simulink model "A01274570_ACT_MATLAB_ROBOTDK"  (R2022a)
settings: Solver=ode45  StartTime=0.0  StopTime=60  MaxStep=.2  RelTol=1e-3  EnableMultiTasking=on
PreLoadFcn:
  | clear all
settings Model: Creator=Student  LastModifiedBy=osher
settings SolverCC: AlgebraicLoopSolver=TrustRegion
settings DataIOCC: LimitDataPoints=on  SaveFormat=Array  ReturnWorkspaceOutputs=off
settings OptimizationCC: LifeSpan=inf
settings DebuggingCC: UnconnectedInputMsg=warning  UnconnectedOutputMsg=warning  UnconnectedLineMsg=warning  SFUnexpectedBacktrackingDiag=warning  SFNoUnconditionalDefaultTransitionDiag=warning  SFExecutionAtInitializationDiag=none  SFMachineParentedDataDiag=warning  ArithmeticOperatorsInVariantConditions=warning
settings HardwareCC: ProdBitPerPointer=32  ProdBitPerSizeT=32  ProdBitPerPtrDiffT=32  ProdLargestAtomicFloat=None  ProdIntDivRoundTo=Undefined  ProdEndianess=Unspecified  ProdWordSize=32  ProdHWDeviceType=32-bit Generic
settings ModelReferenceCC: PropagateSignalLabelsOutOfModel=off
settings SFSimCC: SimUseLocalCustomCode=off  CustomCodeUndefinedFunction=UseInterfaceOnly
settings RTWCC: RTWUseLocalCustomCode=off
settings CodeAppCC: StateflowObjectComments=on
settings GRTTargetCC: TargetLangStandard=C89/C90 (ANSI)
settings ConfigComp: CovMetricSettings=dw  CovSaveCumulativeToWorkspaceVar=on  CovSaveSingleToWorkspaceVar=on  CovExternalEMLEnable=off

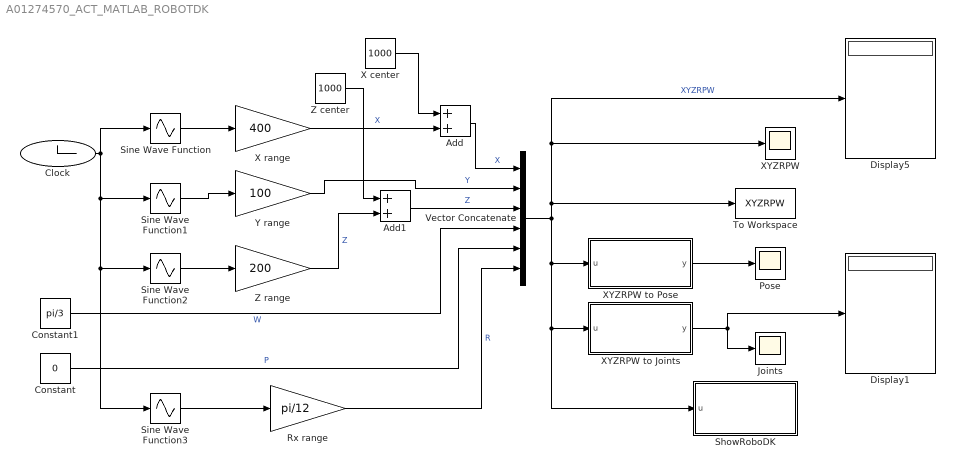
== system A01274570_ACT_MATLAB_ROBOTDK ==
  Add : Sum
  Add1 : Sum
  Clock : Clock
      settings: Decimation=30
  Constant : Constant  Value=0
  Constant1 : Constant  Value=pi/3
  Display1 : Display
  Display5 : Display
  Joints : Scope
  Pose : Scope
  "Rx range " : Gain  Gain=pi/12
  ShowRoboDK : MATLAB Function  TreatAsAtomicUnit=on
  Sine Wave Function : Sin  TimeSource=Use external signal  Frequency=3.1416/32  Phase=3.1416/2  SampleTime=0
  Sine Wave Function1 : Sin  TimeSource=Use external signal  Frequency=3.1416/6  SampleTime=0
  Sine Wave Function2 : Sin  TimeSource=Use external signal  Frequency=3.1416/16  Phase=3.1416  SampleTime=0
  Sine Wave Function3 : Sin  TimeSource=Use external signal  Frequency=3.1416/32  Phase=pi/2  SampleTime=0
  To Workspace : ToWorkspace  VariableName=XYZRPW  SaveFormat=Timeseries  SampleTime=-1
  Vector Concatenate : Concatenate  NumInputs=6
  "X center " : Constant  Value=1000
  X range : Gain  Gain=400
  "XYZRPW " : Scope
  "XYZRPW to Joints " : MATLAB Function  InitFcn="\"ABB IRB 2600-20/1.65\""  TreatAsAtomicUnit=on
  XYZRPW to Pose : MATLAB Function  TreatAsAtomicUnit=on
  Y range : Gain  Gain=100
  "Z center " : Constant  Value=1000
  Z range : Gain  Gain=200
  wires:
  Vector Concatenate/1 -> "XYZRPW "/1, Display5/1, To Workspace/1, ShowRoboDK/1(u), "XYZRPW to Joints "/1(u), XYZRPW to Pose/1(u)  "XYZRPW"
  Clock/1 -> Sine Wave Function3/1, Sine Wave Function2/1, Sine Wave Function1/1, Sine Wave Function/1
  Sine Wave Function/1 -> X range/1
  Sine Wave Function1/1 -> Y range/1
  Sine Wave Function2/1 -> Z range/1
  Sine Wave Function3/1 -> "Rx range "/1
  Add/1 -> Vector Concatenate/1  "X"
  Y range/1 -> Vector Concatenate/2  "Y"
  Add1/1 -> Vector Concatenate/3  "Z"
  "Rx range "/1 -> Vector Concatenate/6  "R"
  Constant/1 -> Vector Concatenate/5  "P"
  Constant1/1 -> Vector Concatenate/4  "W"
  XYZRPW to Pose/1(y) -> Pose/1
  "XYZRPW to Joints "/1(y) -> Joints/1, Display1/1
  Z range/1 -> Add1/2  "Z"
  X range/1 -> Add/2  "X"
  "Z center "/1 -> Add1/1
  "X center "/1 -> Add/1

== matlab function A01274570_ACT_MATLAB_ROBOTDK/XYZRPW to Pose ==
  data: u input; y output
function y = fcn(u)
%#codegen

y = XYZRPW_2_Pose(u);

== matlab function A01274570_ACT_MATLAB_ROBOTDK/ShowRoboDK ==
  data: u input
function fcn(u)
coder.extrinsic('RoboDK_ShowPose');

pose = XYZRPW_2_Pose(u);

RoboDK_ShowPose(pose)

== matlab function A01274570_ACT_MATLAB_ROBOTDK/XYZRPW to Joints  ==
  data: u input; y output
function y = fcn(u)
coder.extrinsic('RoboDK_Pose2Joints');

pose = XYZRPW_2_Pose(u);

joints = zeros(6,1);
joints = RoboDK_Pose2Joints(pose);

y = joints;
